simulink library "r2dbe_vdif_lib"  (R2012b)
settings: Solver=ode45  StartTime=0.0  StopTime=10.0  RelTol=1e-3
libraries: xbsIndex_r4 x3
settings Model: Creator=rprimian  LastModifiedBy=lvertats

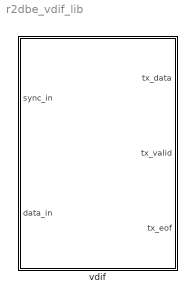
== system r2dbe_vdif_lib ==
  vdif : Subsystem  mask(r2dbe_vdif){}
      mask help: Sub-system for VDIF parameters of the R2DBE.

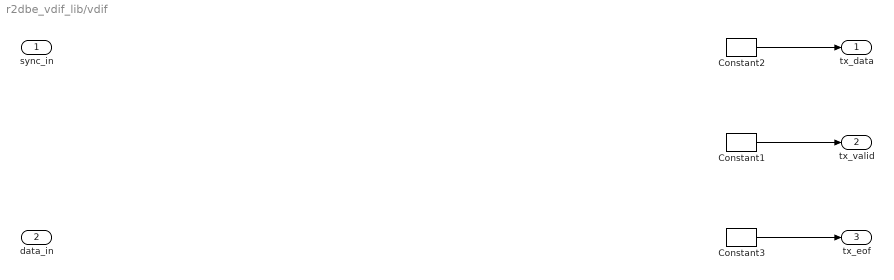
== system r2dbe_vdif_lib/vdif ==
  sync_in : Inport
  data_in : Inport  Port=2
  Constant1 : xbsIndex_r4/Constant  const=0  gui_display_data_type=Boolean  arith_type=Boolean  n_bits=64  bin_pt=0  preci_type=Single  exp_width=8  frac_width=24  explicit_period=on  period=1  equ=P=C  opselect=C  inp2=PCIN>>17  opr=+  inp1=P  carry=CIN  dbl_ovrd=off  block_type=constant
  Constant2 : xbsIndex_r4/Constant  const=0  gui_display_data_type=Fixed-point  arith_type=Unsigned  n_bits=64  bin_pt=0  preci_type=Single  exp_width=8  frac_width=24  explicit_period=on  period=1  equ=P=C  opselect=C  inp2=PCIN>>17  opr=+  inp1=P  carry=CIN  dbl_ovrd=off  block_type=constant
  Constant3 : xbsIndex_r4/Constant  const=0  gui_display_data_type=Boolean  arith_type=Boolean  n_bits=64  bin_pt=0  preci_type=Single  exp_width=8  frac_width=24  explicit_period=on  period=1  equ=P=C  opselect=C  inp2=PCIN>>17  opr=+  inp1=P  carry=CIN  dbl_ovrd=off  block_type=constant
  tx_data : Outport
  tx_valid : Outport  Port=2
  tx_eof : Outport  Port=3
  wires:
  Constant3/1 -> tx_eof/1
  Constant1/1 -> tx_valid/1
  Constant2/1 -> tx_data/1
